simulink model "IndustrialMicrogrid"  (R2023a)
settings: Solver=FixedStepDiscrete  StartTime=0.0  StopTime=10  FixedStep=Ts  RelTol=1e-3
PostLoadFcn:
  | IndustrialMicrogridInputData
  | GfmGridFormingConverterInputParameters
model workspace (MAT data in the model file):
  caseNum = 2
undefined symbols (not defined in the file): base, BESS, DiscIntNeverNeededParam, grid, Grid, gridInverter, machine, microgrid, PV, PVInverter, PVTransformer, scrFactorRg, scrFactorXg, transformer, Ts
libraries: ee_lib x112, eeGeneralControl x104, nesl_utility_internal x64, simulink x56, nesl_utility x37, fl_lib x29, slpidlib x13, eeTransforms x11, eeTotalHarmonicDistorsion x8, eeRmsMeasurement x4, eeSinusoidalMeasurement x4, simulink_extras x2
(part 5 of 14)

== system IndustrialMicrogrid/MG1 Primary Substation/Microgrid Controller/Breaker Control ==
  Bus Element In1 : Inport  PortName=Control Room  Element=ResynchCmd
  Bus Element In4 : Inport  PortName=Control Room  Element=BRKcontrol
  Bus Element In6 : Inport  PortName=Control Room  Element=BRKcontrol
  Bus Element In3 : Inport  PortName=Control Room  Element=PlannedIslandCmd
  Bus Element In5 : Inport  Port=2  PortName=MGController  Element=IslandMGController.MGPlannedIsland.plannedisland
  Bus Element In2 : Inport  Port=2  PortName=MGController  Element=ResynchMGController.MGResynch.resynch
  Cast To Double1 : DataTypeConversion  OutDataTypeStr=double  SaturateOnIntegerOverflow=off  RndMeth=Floor
  Logical Operator1 : Logic  Operator=NOT  AllPortsSameDT=off  OutDataTypeStr=boolean
  Logical Operator{2..5} (4 alike) : Logic  AllPortsSameDT=off  OutDataTypeStr=boolean
  Logical Operator6 : Logic  Operator=OR  AllPortsSameDT=off  OutDataTypeStr=boolean
  Logical Operator7 : Logic  Operator=NOT  AllPortsSameDT=off  OutDataTypeStr=boolean
  BreakerControl : Outport
  wires:
  Logical Operator7/1 -> Logical Operator5/1
  Logical Operator1/1 -> Logical Operator4/1
  Logical Operator5/1 -> Logical Operator6/2
  Logical Operator3/1 -> Logical Operator4/2
  Bus Element In6/1 -> Logical Operator1/1
  Logical Operator6/1 -> Cast To Double1/1
  Bus Element In5/1 -> Logical Operator3/2
  Bus Element In4/1 -> Logical Operator5/2
  Logical Operator4/1 -> Logical Operator6/1
  Bus Element In1/1 -> Logical Operator2/1
  Logical Operator2/1 -> Logical Operator7/1
  Cast To Double1/1 -> BreakerControl/1
  Bus Element In3/1 -> Logical Operator3/1
  Bus Element In2/1 -> Logical Operator2/2

== system IndustrialMicrogrid/MG1 Primary Substation/Microgrid Controller/Frequency Reference ==
  Bus Element In : Inport  PortName=Control Room  Element=ResynchCmd
  Bus Element In1 : Inport  PortName=Control Room  Element=PowerCmd
  Bus Element In4 : Inport  PortName=Control Room  Element=BlackStartMG1
  Bus Element In2 : Inport  Port=2  PortName=MGController  Element=ResynchMGController.MGResynch.synchfrequency
  Bus Element In3 : Inport  Port=2  PortName=MGController  Element=BlackStart.Fref1
  Constant : Constant  Value=IslandFrequency
  Constant1 : Constant  Value=GridFrequency
  Gain1 : Gain  Gain=1/60
  Sum : Sum  Inputs=|++
  Switch : Switch  Criteria=u2 > Threshold  Threshold=0.5  SaturateOnIntegerOverflow=off  InputSameDT=off
  Switch1 : Switch  Criteria=u2 > Threshold  Threshold=0.5  SaturateOnIntegerOverflow=off  InputSameDT=off
  Switch2 : Switch  Criteria=u2 > Threshold  Threshold=0.5  SaturateOnIntegerOverflow=off  InputSameDT=off
  fref : Outport
  wires:
  Bus Element In/1 -> Switch/2
  Switch2/1 -> Switch1/3
  Bus Element In2/1 -> Sum/1
  Switch1/1 -> Gain1/1
  Bus Element In3/1 -> Switch1/1
  Gain1/1 -> fref/1
  Bus Element In4/1 -> Switch1/2
  Bus Element In1/1 -> Switch2/2
  Constant/1 -> Switch/3, Sum/2
  Sum/1 -> Switch/1
  Constant1/1 -> Switch2/1
  Switch/1 -> Switch2/3

== system IndustrialMicrogrid/MG1 Primary Substation/Microgrid Controller/PLL ==
  In Bus Element : Inport  PortName=mPCC  Element=Grid voltage
  In Bus Element1 : Inport  PortName=mPCC  Element=mPCC.voltage
  PLL : Subsystem
  PLL start at 0.2 s : Subsystem
  PLL starts at 0.2 s : Subsystem
  PLL1 : Subsystem
  Bus Element Out : Outport  PortName=Grid  Element=frequency
  Bus Element Out1 : Outport  PortName=Grid  Element=angle
  Bus Element Out2 : Outport  PortName=Grid  Element=voltage
  Bus Element Out3 : Outport  Port=2  PortName=Island  Element=voltage
  Bus Element Out4 : Outport  Port=2  PortName=Island  Element=frequency
  Bus Element Out5 : Outport  Port=2  PortName=Island  Element=angle
  wires:
  In Bus Element/1 -> PLL start at 0.2 s/1(PCC measurement)
  PLL starts at 0.2 s/1(abc) -> PLL1/1(abc)
  In Bus Element1/1 -> PLL starts at 0.2 s/1(PCC measurement)
  PLL start at 0.2 s/1(Out1) -> PLL/1(abc)
  PLL/1(fre) -> Bus Element Out/1
  PLL/2(angle) -> Bus Element Out1/1
  PLL/3(mag) -> Bus Element Out2/1
  PLL1/1(fre) -> Bus Element Out4/1
  PLL1/2(angle) -> Bus Element Out5/1
  PLL1/3(mag) -> Bus Element Out3/1

== system IndustrialMicrogrid/MG1 Primary Substation/Microgrid Controller/Planned Island ==
  mPCCPLL : Inport
  Control Room : Inport  Port=2
  Bus Creator : BusCreator  Inputs=2
  Control for Zero Powerflow : Subsystem  mask(Planned Island Control){KpPPlannedIsland=microgrid.KpPPlannedIsland, KiPPlannedIsland=microgrid.KiPPlannedIsland, KpQPlannedIsland=microgrid.KpQPlannedIsland, KiQPlannedIsland=microgrid.KiQPlannedIsland, ZeroActivePowerThreshold=microgrid.zeroActivePowerThreshold, ZeroReactivePowerThreshold=microgrid.zeroReactivePowerThreshold, PlannedIslandDelay=microgrid.plannedIslandDelay}
      mask prompts: KpPPlannedIsland "Active Power Planned Island Proportional Gain"; KiPPlannedIsland "Active Power Planned Island Integral Gain"; KpQPlannedIsland "Reactive Power Planned Island Proportional Gain"; KiQPlannedIsland "Reactive Power Planned Island Intergal Gain"; ZeroActivePowerThreshold "Zero Active Power Threshold"; ZeroReactivePowerThreshold "Zero Reactive Power Threshold"; PlannedIslandDelay "Planned Island Delay"
      mask help: provide planned island control parameters
  IslandMGController : Outport
  wires:
  mPCCPLL/1 -> Bus Creator/2, Control for Zero Powerflow/2(mPCCPLL)  "PCC measurments"
  Control for Zero Powerflow/1(MGController) -> Bus Creator/1  "MGPlannedIsland"
  Bus Creator/1 -> IslandMGController/1  "IslandMGController"
  Control Room/1 -> Control for Zero Powerflow/1(ControlRoom)

== system IndustrialMicrogrid/MG1 Primary Substation/Microgrid Controller/Resynchronization ==
  Control Room : Inport
  mPCCPLL : Inport  Port=2
  BESS : Inport  Port=3
  Bus Creator : BusCreator  Inputs=2
  Frequency and voltage matching : Subsystem  mask(Resynchronization Control){GridFrequency=grid.frequency, RadToDegree=microgrid.radToDegree, KpFreResynch=microgrid.KpFreResynch, KiFreResynch=microgrid.KiFreResynch, KpVolResynch=microgrid.KpVolResynch, KiVolResynch=microgrid.KiVolResynch, KpAngResynch=microgrid.KpAngResynch, KiAngResynch=microgrid.KiAngResynch, FrequencyThreshold=microgrid.frequencyThreshold, AngleThreshold=microgrid.angleThreshold, VoltageThreshold=microgrid.voltageThreshold, ResynchDelay=microgrid.resynchDelay, kDroop=microgrid.KDroop}
      mask prompts: GridFrequency "Grid Frequency"; RadToDegree "Rad to Degree"; KpFreResynch "Frequency Resynch Proportional Gain"; KiFreResynch "Frequency Resynch Integral Gain"; KpVolResynch "Voltage Resynch Proportional Gain"; KiVolResynch "Voltage Resynch Integral Gain"; KpAngResynch "Angle Resynch Proportional Gain"; KiAngResynch "Angle Resynch Integral Gain"; FrequencyThreshold "Frequency Matching Threshold"; AngleThreshold "Angle Matching Threshold"; VoltageThreshold "Voltage Matching Threshold"; ResynchDelay "Resynch Delay"; kDroop "Voltage Droop"
      mask help: Provide input for resynchronization control parameters
  ResynchMGController : Outport
  wires:
  Control Room/1 -> Frequency and voltage matching/2(ControlRoom)
  Bus Creator/1 -> ResynchMGController/1  "ResynchMGController"
  Frequency and voltage matching/1(MGController) -> Bus Creator/1  "MGResynch"
  BESS/1 -> Frequency and voltage matching/1(BESS)
  mPCCPLL/1 -> Bus Creator/2, Frequency and voltage matching/3(mPCCPLL)  "PCC measurments"

== system IndustrialMicrogrid/MG1 Primary Substation/Microgrid Controller/Voltage Reference ==
  Bus Element In1 : Inport  PortName=Control Room  Element=ResynchCmd
  Bus Element In2 : Inport  PortName=Control Room  Element=BlackStartMG1
  Bus Element In3 : Inport  Port=2  PortName=MGController  Element=ResynchMGController.MGResynch.synchvoltagedpr
  Bus Element In4 : Inport  Port=2  PortName=MGController  Element=BlackStart.Vref1
  Constant9 : Constant  Value=IslandVoltage
  Switch1 : Switch  Criteria=u2 > Threshold  Threshold=0.5  SaturateOnIntegerOverflow=off  InputSameDT=off
  Switch2 : Switch  Criteria=u2 > Threshold  Threshold=0.5  SaturateOnIntegerOverflow=off  InputSameDT=off
  Vref : Outport
  wires:
  Switch2/1 -> Vref/1
  Switch1/1 -> Switch2/3
  Bus Element In2/1 -> Switch2/2
  Constant9/1 -> Switch1/3
  Bus Element In1/1 -> Switch1/2
  Bus Element In4/1 -> Switch2/1
  Bus Element In3/1 -> Switch1/1

== system IndustrialMicrogrid/MG1 Primary Substation/PCC Measurements and PCC Breaker/Grid Current Measurement ==
  Current and Voltage Sensor (Three-Phase)1 : ee_lib/Sensors & Transducers/Current and Voltage Sensor (Three-Phase)  vMeasurementType=ee.enum.vmeasurement.ll  outputUnit=ee.enum.unit.pu  SRated=2.5e6 A*V  VRated=microgrid.voltage V  I_specify=off  I_priority=None  I=[0, 0, 0] A  I_nominal_specify=off  I_nominal_unit=A  I_nominal_value=1  V_specify=off  V_priority=None  V=[0, 0, 0] V  V_nominal_specify=off  V_nominal_unit=V  V_nominal_value=1
      settings: InternalSimscapePortConfiguration="{\"Bottom\":[],\"Left\":[{\"id\":\"N1\",\"label\":\"~1\",\"type\":\"foundation.electrical.three_phase\"}],\"Right\":[{\"id\":\"V_output\",\"label\":\"V\",\"type\":\"output\"},{\"id\":\"I_output\",\"label\":\"I\",\"type\":\"output\"},{\"id\":\"N2\",\"label\":\"~2\",\"type\":\"foundation.electrical.three_phase\"}],\"Top\":[]}"
  PS-Simulink Converter2 : nesl_utility_internal/PS-Simulink Converter  PhysicalDomain=network_engine_domain  SubClassName=ps_output  LeftPortType=input  RightPortType=output  PseudoPeriodic=off  Frequencies=[]  VectorFormat=1-D array  Unit=V  AffineConversion=off
  PS-Simulink Converter3 : nesl_utility_internal/PS-Simulink Converter  PhysicalDomain=network_engine_domain  SubClassName=ps_output  LeftPortType=input  RightPortType=output  PseudoPeriodic=off  Frequencies=[]  VectorFormat=1-D array  Unit=A  AffineConversion=off
  Terminator : Terminator
  ~ : PMIOPort  Side=Left
  "~ " : PMIOPort  Port=2  Side=Right
  "Grid voltage " : Outport
  wires:
  PS-Simulink Converter2/1 -> "Grid voltage "/1
  PS-Simulink Converter3/1 -> Terminator/1
  connections:
  Current and Voltage Sensor (Three-Phase)1/RConn1 -- PS-Simulink Converter2/LConn1
  ~/RConn1 -- Current and Voltage Sensor (Three-Phase)1/LConn1
  Current and Voltage Sensor (Three-Phase)1/RConn2 -- PS-Simulink Converter3/LConn1
  Current and Voltage Sensor (Three-Phase)1/RConn3 -- "~ "/RConn1

== system IndustrialMicrogrid/MG1 Primary Substation/PCC Measurements and PCC Breaker/Grid Power Measurement ==
  Current and Voltage Sensor (Three-Phase) : ee_lib/Sensors & Transducers/Current and Voltage Sensor (Three-Phase)  vMeasurementType=ee.enum.vmeasurement.ll  outputUnit=ee.enum.unit.pu  SRated=2.5e6 A*V  VRated=microgrid.voltage V  I_specify=off  I_priority=None  I=[0, 0, 0] A  I_nominal_specify=off  I_nominal_unit=A  I_nominal_value=1  V_specify=off  V_priority=None  V=[0, 0, 0] V  V_nominal_specify=off  V_nominal_unit=V  V_nominal_value=1
      settings: InternalSimscapePortConfiguration="{\"Bottom\":[],\"Left\":[{\"id\":\"N1\",\"label\":\"~1\",\"type\":\"foundation.electrical.three_phase\"}],\"Right\":[{\"id\":\"V_output\",\"label\":\"V\",\"type\":\"output\"},{\"id\":\"I_output\",\"label\":\"I\",\"type\":\"output\"},{\"id\":\"N2\",\"label\":\"~2\",\"type\":\"foundation.electrical.three_phase\"}],\"Top\":[]}"
  Low-Pass Filter (Discrete or Continuous) : eeGeneralControl/Low-Pass Filter (Discrete or Continuous)  K=1  T=0.1  B=inf  A=-inf  init_option=Inherited from block input  x0=0  Ts=Ts
  Low-Pass Filter (Discrete or Continuous)1 : eeGeneralControl/Low-Pass Filter (Discrete or Continuous)  K=1  T=0.1  B=inf  A=-inf  init_option=Inherited from block input  x0=0  Ts=Ts
  PS-Simulink Converter : nesl_utility_internal/PS-Simulink Converter  PhysicalDomain=network_engine_domain  SubClassName=ps_output  LeftPortType=input  RightPortType=output  PseudoPeriodic=off  Frequencies=[]  VectorFormat=1-D array  Unit=inherit  AffineConversion=off
  PS-Simulink Converter1 : nesl_utility_internal/PS-Simulink Converter  PhysicalDomain=network_engine_domain  SubClassName=ps_output  LeftPortType=input  RightPortType=output  PseudoPeriodic=off  Frequencies=[]  VectorFormat=1-D array  Unit=inherit  AffineConversion=off
  PS-Simulink Converter8 : nesl_utility_internal/PS-Simulink Converter  PhysicalDomain=network_engine_domain  SubClassName=ps_output  LeftPortType=input  RightPortType=output  PseudoPeriodic=off  Frequencies=[]  VectorFormat=1-D array  Unit=MW  AffineConversion=off
  PS-Simulink Converter9 : nesl_utility_internal/PS-Simulink Converter  PhysicalDomain=network_engine_domain  SubClassName=ps_output  LeftPortType=input  RightPortType=output  PseudoPeriodic=off  Frequencies=[]  VectorFormat=1-D array  Unit=MV*A  AffineConversion=off
  Power Sensor (Three-Phase)2 : ee_lib/Sensors & Transducers/Power Sensor (Three-Phase)  load_type=ee.enum.passive.type_balanced.balanced  f0=60 Hz  config=ee.enum.with_neutral.no  rho=1
      settings: InternalSimscapePortConfiguration="{\"Bottom\":[],\"Left\":[{\"id\":\"N1\",\"label\":\"~1\",\"type\":\"foundation.electrical.three_phase\"}],\"Right\":[{\"id\":\"N2\",\"label\":\"~2\",\"type\":\"foundation.electrical.three_phase\"}],\"Top\":[{\"id\":\"Pm\",\"label\":\"P\",\"type\":\"output\"},{\"id\":\"Qm\",\"label\":\"Q\",\"type\":\"output\"}]}"
  ~ : PMIOPort  Side=Left
  "~ " : PMIOPort  Port=2  Side=Right
  Out Bus Element : Outport  PortName=mPCC  Element=voltage
  Out Bus Element1 : Outport  PortName=mPCC  Element=current
  Out Bus Element2 : Outport  PortName=mPCC  Element=activepower
  Out Bus Element3 : Outport  PortName=mPCC  Element=reactivepower
  wires:
  PS-Simulink Converter8/1 -> Low-Pass Filter (Discrete or Continuous)/1
  PS-Simulink Converter9/1 -> Low-Pass Filter (Discrete or Continuous)1/1
  PS-Simulink Converter/1 -> Out Bus Element/1
  PS-Simulink Converter1/1 -> Out Bus Element1/1
  Low-Pass Filter (Discrete or Continuous)/1 -> Out Bus Element2/1
  Low-Pass Filter (Discrete or Continuous)1/1 -> Out Bus Element3/1
  connections:
  Current and Voltage Sensor (Three-Phase)/RConn2 -- PS-Simulink Converter1/LConn1
  PS-Simulink Converter/LConn1 -- Current and Voltage Sensor (Three-Phase)/RConn1
  Power Sensor (Three-Phase)2/RConn1 -- Current and Voltage Sensor (Three-Phase)/LConn1
  PS-Simulink Converter9/LConn1 -- Power Sensor (Three-Phase)2/LConn3
  Current and Voltage Sensor (Three-Phase)/RConn3 -- "~ "/RConn1
  PS-Simulink Converter8/LConn1 -- Power Sensor (Three-Phase)2/LConn2
  ~/RConn1 -- Power Sensor (Three-Phase)2/LConn1

== system IndustrialMicrogrid/MG2 PV Plant/(500KWp PV)/Measurement2 ==
  u : Inport
  Lead-Lag (Discrete or Continuous) : eeGeneralControl/Lead-Lag (Discrete or Continuous)  T1=0  T2=PV.controllerTSensor  B=inf  A=-inf  init_option=Inherited from block input  x0=0  Ts=Ts
      settings: LibrarySourceBlock=|
      | ee_sl_lib/General Control/Lead-Lag
      | (Discrete or Continuous)
  Out Bus Element : Outport  PortName=ipv1  Element=1
  wires:
  Lead-Lag (Discrete or Continuous)/1 -> Out Bus Element/1
  u/1 -> Lead-Lag (Discrete or Continuous)/1

== system IndustrialMicrogrid/MG2 PV Plant/(500KWp PV)/PV Inverter A2 ==
  note: Voltage reference for the PV inverter
  Insolation : Inport
  In Bus Element : Inport  Port=2  PortName=Vbus
  In Bus Element2 : Inport  Port=3  PortName=LVRT
  In Bus Element1 : Inport  Port=4  PortName=ipv1
  Q_ref : Inport  Port=5
  PV & Inverter : Subsystem
  PV Controller : Subsystem
  abc : PMIOPort  Side=Right
  wires:
  Q_ref/1 -> PV Controller/5(Q_ref)
  PV Controller/1(m_abc) -> [m]
  In Bus Element1/1 -> PV Controller/2(ipv1)
  PV & Inverter/1(PV_plant1) -> PV Controller/1(PV_plant1)
  In Bus Element/1 -> PV Controller/4(Vbus)
  In Bus Element2/1 -> PV Controller/3(LVRT)
  [m] -> PV & Inverter/2(reference)
  Insolation/1 -> PV & Inverter/1(Solar insolation)
  connections:
  abc/RConn1 -- PV & Inverter/RConn1

== system IndustrialMicrogrid/MG2 PV Plant/PLL & Measurements2/Measurement2 ==
  u : Inport
  Lead-Lag Filter1 : spsLeadLagFilterLib/Lead-Lag Filter  T1=0  T2=PV.controllerTSensor  Vdc_Init=0  Ts=Ts
  Vg : Outport
  wires:
  Lead-Lag Filter1/1 -> Vg/1
  u/1 -> Lead-Lag Filter1/1

== system IndustrialMicrogrid/MG2 PV Plant/PLL & Measurements2/PLL ==
  abc : Inport
  Demux : Demux  Outputs=3
  Park Transform : eeTransforms/Park Transform  AxisAlignment=Q-axis  PowerInvariant=off
  "Sinusoidal Measurement (PLL, Three-Phase)" : eeSinusoidalMeasurementV2/Sinusoidal Measurement (PLL, Three-Phase)  Kp_LF=PV.kpPLL  Ki_LF=PV.kiPLL  F0=60  Theta0=0  Ts=-1
      settings: LibrarySourceBlock=|
      | ee_sl_lib/Measurements/Sinusoidal Measurement
      | (PLL, Three-Phase)
  Terminator : Terminator
  mag : Outport
  freq : Outport  Port=2
  angle : Outport  Port=3
  Vd : Outport  Port=4
  Vq : Outport  Port=5
  wires:
  Demux/3 -> Terminator/1
  abc/1 -> Park Transform/1, "Sinusoidal Measurement (PLL, Three-Phase)"/1
  Park Transform/1 -> Demux/1
  Demux/1 -> Vd/1
  Demux/2 -> Vq/1
  "Sinusoidal Measurement (PLL, Three-Phase)"/2 -> Park Transform/2, angle/1
  "Sinusoidal Measurement (PLL, Three-Phase)"/1 -> freq/1
  "Sinusoidal Measurement (PLL, Three-Phase)"/3 -> mag/1

== system IndustrialMicrogrid/MG2 Power Center/Diesel Generator/AVR and Exciter ==
  Constant{3,5..9} (6 alike) : Constant  Value=0
  Constant4 : Constant  Value=1.08
  "E_FD Simulink-PS " : nesl_utility/Simulink-PS Converter  PhysicalDomain=network_engine_domain  SubClassName=ps_input  LeftPortType=input  RightPortType=output  PseudoPeriodic=off  Frequencies=[]  NoiseDistribution=none  NoiseParameters=[]  Unit=1  AffineConversion=off  FilteringAndDerivatives=provide  SimscapeFilterOrder=1  InputFilterTimeConstant=.001  UdotUserProvided=0
  I_FD PS-Simulink : nesl_utility/PS-Simulink Converter  PhysicalDomain=network_engine_domain  SubClassName=ps_output  LeftPortType=input  RightPortType=output  PseudoPeriodic=off  Frequencies=[]  VectorFormat=1-D array  Unit=1  AffineConversion=off
  SM DC2C : eeSmDC2C/SM DC2C  E_FD0=1  Ts=-1  R_C=0  X_C=0  T_R=0  K_A=300  T_A=0.06  T_B=0  T_C=0  K_F=0.058  T_F=0.62  V_Rmax=4.5  V_Rmin=-4.5  oelInputLocation=Unused  uelInputLocation=Unused  sclInputLocation=Unused  K_E=1  T_E=1.33  E_FDmin=-99  E_1=3.05  S_E_E1=0.279  E_2=2.29  S_E_E2=0.117
  Synchronous Machine Field Circuit (pu) : ee_lib/Electromechanical/Synchronous/Synchronous Machine Field Circuit  unit_option=ee.enum.unit.pu  SRated=microgrid.dieselRatedPower V*A  FRated=microgrid.frequency Hz  fieldCircuitParameterization_option=ee.enum.sm.fieldparameterization.current  baseEfd=200 V  baseIfd=1300 A  parameterization_option=2  Ladu=1.66  Rfd=0.0006  Xl=0.05  Xd=1.72  Xdd=0.13  Xddd=0.09  d_option=ee.enum.circuit.open  Td0d=0.75 s  Tdd=0.03 s  Td0dd=0.003 s  Tddd=0.008 s
      settings: InternalSimscapePortConfiguration="{\"Bottom\":[],\"Left\":[{\"id\":\"Efd_pu\",\"label\":\"Efd_pu\",\"type\":\"input\"},{\"id\":\"Ifd_pu\",\"label\":\"Ifd_pu\",\"type\":\"output\"}],\"Right\":[{\"id\":\"fd_p\",\"label\":\"fd+\",\"type\":\"foundation.electrical.electrical\"},{\"id\":\"fd_n\",\"label\":\"fd-\",\"type\":\"foundation.electrical.electrical\"}],\"Top\":[]}"
  Terminal Current Measurement : ee_lib/Electromechanical/Synchronous/Synchronous Machine Measurement  output_idx=15
      settings: InternalSimscapePortConfiguration="{\"Bottom\":[],\"Left\":[{\"id\":\"pu_input\",\"label\":\"pu\",\"type\":\"input\"}],\"Right\":[{\"id\":\"pu_output\",\"label\":\"o\",\"type\":\"output\"}],\"Top\":[]}"
  Terminal Current PS-Simulink : nesl_utility/PS-Simulink Converter  PhysicalDomain=network_engine_domain  SubClassName=ps_output  LeftPortType=input  RightPortType=output  PseudoPeriodic=off  Frequencies=[]  VectorFormat=1-D array  Unit=1  AffineConversion=off
  Terminal Voltage Measurement : ee_lib/Electromechanical/Synchronous/Synchronous Machine Measurement  output_idx=14
      settings: InternalSimscapePortConfiguration="{\"Bottom\":[],\"Left\":[{\"id\":\"pu_input\",\"label\":\"pu\",\"type\":\"input\"}],\"Right\":[{\"id\":\"pu_output\",\"label\":\"o\",\"type\":\"output\"}],\"Top\":[]}"
  Terminal Voltage PS-Simulink : nesl_utility/PS-Simulink Converter  PhysicalDomain=network_engine_domain  SubClassName=ps_output  LeftPortType=input  RightPortType=output  PseudoPeriodic=off  Frequencies=[]  VectorFormat=1-D array  Unit=1  AffineConversion=off
  Terminator : Terminator
  Unit Delay : UnitDelay  InitialCondition=1.32943  SampleTime=-1  HasFrameUpgradeWarning=on
  pu : PMIOPort  Side=Left
  fd+ : PMIOPort  Port=2  Side=Right
  fd- : PMIOPort  Port=3  Side=Right
  wires:
  Terminal Current PS-Simulink/1 -> SM DC2C/4
  SM DC2C/1 -> "E_FD Simulink-PS "/1
  Constant9/1 -> SM DC2C/9
  Constant8/1 -> SM DC2C/8
  Constant7/1 -> SM DC2C/7
  Constant6/1 -> SM DC2C/6
  Constant5/1 -> SM DC2C/5
  Constant4/1 -> SM DC2C/1
  Constant3/1 -> SM DC2C/2
  Terminal Voltage PS-Simulink/1 -> SM DC2C/3
  I_FD PS-Simulink/1 -> Unit Delay/1
  Unit Delay/1 -> Terminator/1
  connections:
  Terminal Current Measurement/RConn1 -- Terminal Current PS-Simulink/LConn1
  Terminal Voltage Measurement/RConn1 -- Terminal Voltage PS-Simulink/LConn1
  pu/RConn1 -- Terminal Current Measurement/LConn1 -- Terminal Voltage Measurement/LConn1
  Synchronous Machine Field Circuit (pu)/RConn1 -- fd+/RConn1
  fd-/RConn1 -- Synchronous Machine Field Circuit (pu)/RConn2
  I_FD PS-Simulink/LConn1 -- Synchronous Machine Field Circuit (pu)/LConn2
  "E_FD Simulink-PS "/RConn1 -- Synchronous Machine Field Circuit (pu)/LConn1

== system IndustrialMicrogrid/MG2 Power Center/Diesel Generator/Governor and Prime Mover  ==
  Governor : Subsystem
  Ideal Torque Source : fl_lib/Mechanical/Mechanical Sources/Ideal Torque Source
  Mechanical Rotational Reference : fl_lib/Mechanical/Rotational Elements/Mechanical Rotational Reference
  Non-reheat turbine : Subsystem
  PS-Simulink Converter : nesl_utility/PS-Simulink Converter  PhysicalDomain=network_engine_domain  SubClassName=ps_output  LeftPortType=input  RightPortType=output  PseudoPeriodic=off  Frequencies=[]  VectorFormat=1-D array  Unit=1  AffineConversion=off
  Rotor Velocity Measurement : ee_lib/Electromechanical/Synchronous/Synchronous Machine Measurement  output_idx=4
      settings: InternalSimscapePortConfiguration="{\"Bottom\":[],\"Left\":[{\"id\":\"pu_input\",\"label\":\"pu\",\"type\":\"input\"}],\"Right\":[{\"id\":\"pu_output\",\"label\":\"o\",\"type\":\"output\"}],\"Top\":[]}"
  Simulink-PS Converter : nesl_utility/Simulink-PS Converter  PhysicalDomain=network_engine_domain  SubClassName=ps_input  LeftPortType=input  RightPortType=output  PseudoPeriodic=off  Frequencies=[]  NoiseDistribution=none  NoiseParameters=[]  Unit=1  AffineConversion=off  FilteringAndDerivatives=zero  SimscapeFilterOrder=1  InputFilterTimeConstant=0.001  UdotUserProvided=1
  scale by base_torque : Gain  Gain=base_torque
  R : PMIOPort  Side=Right
  C : PMIOPort  Port=2  Side=Right
  pu : PMIOPort  Port=3  Side=Left
  wires:
  PS-Simulink Converter/1 -> Governor/1(pu_velocity)
  Governor/1(delta_y) -> Non-reheat turbine/1(delta_y)
  Non-reheat turbine/1(torque) -> scale by base_torque/1
  scale by base_torque/1 -> Simulink-PS Converter/1
  connections:
  C/RConn1 -- Ideal Torque Source/RConn2 -- Mechanical Rotational Reference/LConn1
  Ideal Torque Source/LConn1 -- R/RConn1
  pu/RConn1 -- Rotor Velocity Measurement/LConn1
  PS-Simulink Converter/LConn1 -- Rotor Velocity Measurement/RConn1
  Simulink-PS Converter/RConn1 -- Ideal Torque Source/RConn1

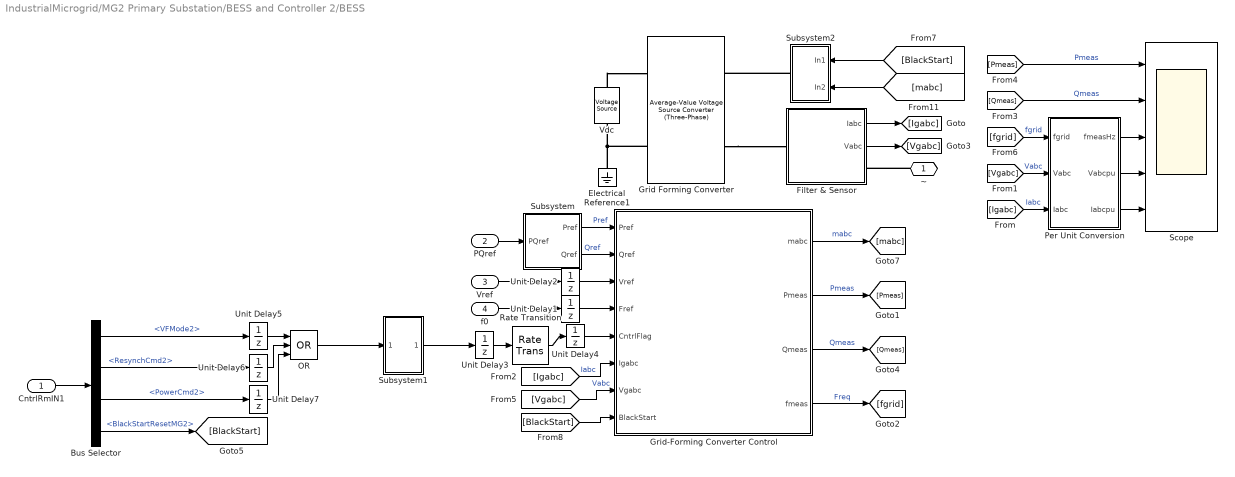
== system IndustrialMicrogrid/MG2 Primary Substation/BESS and Controller 2/BESS ==
  CntrlRmIN1 : Inport
  PQref : Inport  Port=2
  Vref : Inport  Port=3
  f0 : Inport  Port=4
  Bus Selector : BusSelector  OutputSignals=VFMode2,ResynchCmd2,PowerCmd2,BlackStartResetMG2
  Electrical Reference1 : fl_lib/Electrical/Electrical Elements/Electrical Reference
  Filter & Sensor : Subsystem
      mask Display: image('$imagefile'); % Use "Edit Image" on toolstrip to change.
  Grid Forming Converter : ee_lib/Semiconductors & Converters/Converters/Average-Value Voltage Source Converter (Three-Phase)  port_option=ee.enum.threePhasePort.composite  frequency_option=ee.enum.converters.frequency.variable  FRated=50 Hz  losses_parameterization=ee.enum.converters.losses.fixed  Pfixed=1 W  ks=0.01  kc1=1.7 V  kc2=0.01 Ohm  Ploss_vect=[100, 800, 1870, 3250, 4900] W  Irms_vect=[10, 100, 200, 300, 400] A  Vdc_nom=300 V  thermal_mass=30000 J/K  temperature_specify=off  temperature_priority=High  temperature=298.15 K  temperature_nominal_specify=off  temperature_nominal_unit=K  temperature_nominal_value=1
      settings: InternalSimscapePortConfiguration="{\"Bottom\":[],\"Left\":[{\"id\":\"ModWave\",\"label\":\"ModWave\",\"type\":\"input\"},{\"id\":\"N\",\"label\":\"~\",\"type\":\"foundation.electrical.three_phase\"}],\"Right\":[{\"id\":\"p\",\"label\":\"+\",\"type\":\"foundation.electrical.electrical\"},{\"id\":\"n\",\"label\":\"-\",\"type\":\"foundation.electrical.electrical\"}],\"Top\":[]}"
  Grid-Forming Converter Control : Subsystem  mask(Grid Forming Controller){power=gridInverter.apparentPower*1e3, girdLineVoltage=gridInverter.lineRMSVoltage, powerFreq=gridInverter.frequency, dcBusVoltage=gridInverter.DCVoltage, measSampleTime=gridInverter.measurementSampleTime, powerControl=Virtual Synchronous Machine, activePowerSampleTime=gridInverter.droopControl.sampleTime, droopSlope=gridInverter.droopControl.freqSlopeMp, droopT1=gridInverter.droopControl.T1, droopT2=gridInverter.droopControl.T2, droopTC=gridInverter.droopControl.lpfTimeConst, vsmPmeasFilterTC=gridInverter.vsm.PmeasTimeConst, vsmFreqDroop=gridInverter.vsm.freqDroop, vsmInertiaTC=gridInverter.vsm.inertiaConstant, vsmDampingConst=gridInverter.vsm.dampingCoefficent, dampingPowerMaxLimit=gridInverter.vsm.maxDampingPower, dampingPowerMinLimit=gridInverter.vsm.minDampingPower, freqMeasTimeConst=gridInverter.freqMeasTimeConst, freqOption=Constant Frequency Reference, voltreference=gridInverter.Qcontrol.voltageReference, QVoltFilterTC=gridInverter.Qcontrol.QmeasTimeConst, QVoltDroop=gridInverter.Qcontrol.voltageDroop, currentLimit=Virtual Impedance, maxSatCurrentLimit=gridInverter.currentLimit.maxSaturationCurrent, maxVICurrentLimit=gridInverter.currentLimit.viCurrentLimit, ctLimitVirtualImp=gridInverter.currentLimit.virImpResistanceCoeff, ctLimitXbyR=gridInverter.currentLimit.virImpXbyR, ctLimitDelayTime=gridInverter.currentLimit.maxSaturationDelay, currentSatTime=gridInverter.currentLimit.satCurrentRunTime, currentVITimeConst=gridInverter.currentLimit.viFilterTimeConst, voltControlTs=gridInverter.controller.VoltageControlSampleTime, vdPGain=gridInverter.controller.voltControllerKp, VdIGain=gridInverter.controller.voltControllerKi, VdMaxCt=gridInverter.controller.voltageMaxId, VdMinCt=gridInverter.controller.voltageMinId, VqPGain=gridInverter.controller.voltControllerKp, VqIGain=gridInverter.controller.voltControllerKi, VqMaxCt=gridInverter.controller.voltageMaxIq, VqMinCt=gridInverter.controller.voltageMinIq, vdvqLPFTimeConst=gridInverter.controller.voltMeasTimeConst, currentControlTs=gridInverter.controller.CurrentControlSampleTime, filterInductance=gridInverter.L, IdPGain=gridInverter.controller.ctControllerKp, IdIGain=gridInverter.controller.ctControllerKi, IqPGain=gridInverter.controller.ctControllerKp, IqIGain=gridInverter.controller.ctControllerKi}
      mask prompts: power "Grid forming converter power (VA)"; girdLineVoltage "Grid line voltage (V)"; powerFreq "Grid frequency (Hz)"; dcBusVoltage "DC bus voltage"; measSampleTime "Measurement sample time"; powerControl "Active Power Control"; activePowerSampleTime "Sample time (s)"; droopSlope "Power droop slope (pu, Hz/W)"; droopT1 "Lead-Lag numerator time constant (s)"; droopT2 "Lead-Lag denominator time constant (s)"; droopTC "Filter cut-off time constant (s)"; vsmPmeasFilterTC "Power measurement filter time constant (s)"; vsmFreqDroop "Frequency droop (pu,  W/Hz)"; vsmInertiaTC "Inertia constant M (pu)"; vsmDampingConst "Damping constant (pu/Hz)"; dampingPowerMaxLimit "Damping power maximum limit (pu)"; dampingPowerMinLimit "Damping power minimum limit (pu)"; freqMeasTimeConst "Frequency measurement time constant (s)"; freqOption "Damping power fequency option"; voltreference "Voltage reference value (pu)"; QVoltFilterTC "Power measurement filter time constant (s)"; QVoltDroop "Voltage droop (pu, V/VAR)"; currentLimit "Current limiting method"; maxSatCurrentLimit "Maximum current saturation (pu)"; maxVICurrentLimit "Maximum virtual impedance current (pu)"; ctLimitVirtualImp "Virtual impedance coefficient (pu.Ohm/pu.A)"; ctLimitXbyR "Virtual X/R ratio"; ctLimitDelayTime "Maximum current delay time (s)"; currentSatTime "Current limiting run time (s)"; currentVITimeConst "Filter time constant (s)"; voltControlTs "Controller sample time (s)"; vdPGain "Vd proportional gain"; VdIGain "Vd integral gain"; VdMaxCt "Vd maximum current limit (A)"; VdMinCt "Vd minimum current limit (A)"; VqPGain "Vq proportional gain"; VqIGain "Vq integral gain"; VqMaxCt "Vq maximum current limit (A)"; VqMinCt "Vq minimum current limit (A)"; vdvqLPFTimeConst "Voltage measurement filter time constant (s)"; currentControlTs "Controller sample time (s)"; filterInductance "Filter inductance (H)"; IdPGain "Id proportional gain"; IdIGain "Id integral gain"; IqPGain "Iq proportional gain"; IqIGain "Iq integral gain"
      mask help: This block implements the grid forming controller with fault ride through capability. Input to the controller are active and reactive power reference in per unit and the sensed three-phase phase current in amphere and phase voltage in volts.
      mask init: same as IndustrialMicrogrid/MG1 Primary Substation/BESS and Controller/BESS/Grid-Forming Converter Control
      mask TypeOptions powerControl: Virtual Synchronous Machine | Droop Control
      mask Callback powerControl:
      | h = Simulink.Mask.get(gcb);
      | slectedActivePowerControl=get_param(gcb,'powerControl');
      | %slectedActivePowerControl = h.Parameters(find(string({h.Parameters.Name}) == 'powerControl')).Value;
      | switch slectedActivePowerControl
      |     case 'Virtual Synchronous Machine'
      |         h.Parameters(find(string({h.Parameters.Name}) == 'droopSlope')).Visible = 'off';
      |         h.Parameters(find(string({h.Parameters.Name}) == 'droopTC')).Visible = 'off';
      |         h.Parameters(find(string({h.Parameters.Name}) == 'droopT1')).Visible = 'off';
      |         h.Parameters(find(string({h.Parameters.Name}) == 'droopT2')).Visible = 'off';
      |         h.Parameters(find(string({h.Parameters.Name}) == 'vsmPmeasFilterTC')).Visible = 'on';
      |         h.Parameters(find(string({h.Parameters.Name}) == 'vsmFreqDroop')).Visible = 'on';
      |         h.Parameters(find(string({h.Parameters.Name}) == 'vsmInertiaTC')).Visible = 'on';
      |         h.Parameters(find(string({h.Parameters.Name}) == 'vsmDampingConst')).Visible = 'on';
      |         h.Parameters(find(string({h.Parameters.Name}) == 'dampingPowerMaxLimit')).Visible = 'on';
      |         h.Parameters(find(string({h.Parameters.Name}) == 'dampingPowerMinLimit')).Visible = 'on';
      |         h.Parameters(find(string({h.Parameters.Name}) == 'freqOption')).Visible = 'on';
      |         h.Parameters(find(string({h.Parameters.Name}) == 'freqMeasTimeConst')).Visible = 'on';
      |     case 'Droop Control'
      |         h.Parameters(find(string({h.Parameters.Name}) == 'droopSlope')).Visible = 'on';
      |         h.Parameters(find(string({h.Parameters.Name}) == 'droopTC')).Visible = 'on';
      |         h.Parameters(find(string({h.Parameters.Name}) == 'droopT1')).Visible = 'on';
      |         h.Parameters(find(string({h.Parameters.Name}) == 'droopT2')).Visible = 'on';
      |         h.Parameters(find(string({h.Parameters.Name}) == 'vsmPmeasFilterTC')).Visible = 'off';
      |         h.Parameters(find(string({h.Parameters.Name}) == 'vsmFreqDroop')).Visible = 'off';
      |         h.Parameters(find(string({h.Parameters.Name}) == 'vsmInertiaTC')).Visible = 'off';
      |         h.Parameters(find(string({h.Parameters.Name}) == 'vsmDampingConst')).Visible = 'off';
      |         h.Parameters(find(string({h.Parameters.Name}) == 'dampingPowerMaxLimit')).Visible = 'off';
      |         h.Parameters(find(string({h.Parameters.Name}) == 'dampingPowerMinLimit')).Visible = 'off';
      |         h.Parameters(find(string({h.Parameters.Name}) == 'freqOption')).Visible = 'off';
      |         h.Parameters(find(string({h.Parameters.Name}) == 'freqMeasTimeConst')).Visible = 'on';
      | 
      |     otherwise
      |         disp('Choose proper active power control method')
      | end
      mask TypeOptions freqOption: Use Grid Frequency Measurement | Constant Frequency Reference
      mask TypeOptions currentLimit: Virtual Impedance | Current Limiting | Combining Virtual Impedance and Current Limiting
      mask Callback currentLimit:
      | currentLimit = 1;
      | h = Simulink.Mask.get(gcb);
      | currentLimitControl=get_param(gcb,'currentLimit');
      | %slectedActivePowerControl = h.Parameters(find(string({h.Parameters.Name}) == 'powerControl')).Value;
      | switch currentLimitControl
      |     case 'Virtual Impedance'
      |         h.Parameters(find(string({h.Parameters.Name}) == 'maxVICurrentLimit')).Visible = 'on';
      |         h.Parameters(find(string({h.Parameters.Name}) == 'ctLimitVirtualImp')).Visible = 'on';
      |         h.Parameters(find(string({h.Parameters.Name}) == 'ctLimitXbyR')).Visible = 'on';
      |         h.Parameters(find(string({h.Parameters.Name}) == 'maxSatCurrentLimit')).Visible = 'off';
      |         h.Parameters(find(string({h.Parameters.Name}) == 'ctLimitDelayTime')).Visible = 'off';
      |         h.Parameters(find(string({h.Parameters.Name}) == 'currentSatTime')).Visible = 'off';
      |         h.Parameters(find(string({h.Parameters.Name}) == 'currentVITimeConst')).Visible = 'on';
      | 
      | 
      |     case 'Current Limiting'
      |         h.Parameters(find(string({h.Parameters.Name}) == 'maxVICurrentLimit')).Visible = 'off';
      |         h.Parameters(find(string({h.Parameters.Name}) == 'ctLimitVirtualImp')).Visible = 'off';
      |         h.Parameters(find(string({h.Parameters.Name}) == 'ctLimitXbyR')).Visible = 'off';
      |         h.Parameters(find(string({h.Parameters.Name}) == 'maxSatCurrentLimit')).Visible = 'on';
      |         h.Parameters(find(string({h.Parameters.Name}) == 'ctLimitDelayTime')).Visible = 'on';
      |         h.Parameters(find(string({h.Parameters.Name}) == 'currentSatTime')).Visible = 'off';
      |         h.Parameters(find(string({h.Parameters.Name}) == 'currentVITimeConst')).Visible = 'off';
      | 
      |     case 'Combining Virtual Impedance and Current Limiting'
      |         h.Parameters(find(string({h.Parameters.Name}) == 'maxVICurrentLimit')).Visible = 'on';
      |         h.Parameters(find(string({h.Parameters.Name}) == 'ctLimitVirtualImp')).Visible = 'on';
      |         h.Parameters(find(string({h.Parameters.Name}) == 'ctLimitXbyR')).Visible = 'on';
      |         h.Parameters(find(string({h.Parameters.Name}) == 'maxSatCurrentLimit')).Visible = 'on';
      |         h.Parameters(find(string({h.Parameters.Name}) == 'ctLimitDelayTime')).Visible = 'off';
      |         h.Parameters(find(string({h.Parameters.Name}) == 'currentSatTime')).Visible = 'on';
      |         h.Parameters(find(string({h.Parameters.Name}) == 'currentVITimeConst')).Visible = 'on';
      | 
      |     otherwise
      |         disp('Choose proper current limiting method')
      | end
      mask DialogControl ParameterGroupVar Prompt: Grid Forming Control Parameters
      mask DialogControl Container8 Prompt: Grid-forming Converter Specification
      mask DialogControl Pcontrolgrp Prompt: Active Power Controller Parameters
      mask DialogControl QcontrolGrp Prompt: Reactive Power Controller Parameters
      mask DialogControl faultRideThroughGrp Prompt: Fault Ride Through Parameters
      mask DialogControl voltControlgrp Prompt: Voltage Controller Parameters
      mask DialogControl Container15currentContGrp Prompt: Current Controller Parameters
      mask Display: image('$imagefile'); % Use "Edit Image" on toolstrip to change.
  OR : Logic  Operator=OR  Inputs=3  IconShape=distinctive  AllPortsSameDT=off  OutDataTypeStr=boolean
  Per Unit Conversion : Subsystem
  Rate Transition : RateTransition
  Scope : Scope  NumInputPorts=5
  Subsystem : Subsystem
  Subsystem1 : Subsystem
  Subsystem2 : Subsystem
  Unit Delay{1..4} (4 alike) : UnitDelay  InitialCondition=1  SampleTime=Ts  HasFrameUpgradeWarning=on
  Unit Delay5 : UnitDelay  SampleTime=Ts  HasFrameUpgradeWarning=on
  Unit Delay6 : UnitDelay  SampleTime=Ts  HasFrameUpgradeWarning=on
  Unit Delay7 : UnitDelay  SampleTime=Ts  HasFrameUpgradeWarning=on
  Vdc : ee_lib/Sources/Voltage Source  dc_voltage=gridInverter.DCVoltage V  ac_voltage=0 V  ac_shift=0 rad  ac_frequency=0 Hz  noise_mode=ee.enum.sources.noise.Disabled  PSD=0 V^2/Hz  sample_time=1e-3 s  repeatability=ee.enum.sources.repeatability.NotRepeatable  user_seed=0  auto_seed=3499211588  i_specify=off  i_priority=None  i=0 A  i_nominal_specify=off  i_nominal_unit=A  i_nominal_value=1  v_specify=off  v_priority=None  v=0 V  v_nominal_specify=off  v_nominal_unit=V  v_nominal_value=1
  "~ " : PMIOPort  Side=Left
  wires:
  Grid-Forming Converter Control/3(Qmeas) -> [Qmeas]  "Qmeas"
  Grid-Forming Converter Control/2(Pmeas) -> [Pmeas]  "Pmeas"
  Filter & Sensor/2(Vabc) -> [Vgabc]
  Filter & Sensor/1(Iabc) -> [Igabc]
  [Vgabc] -> Grid-Forming Converter Control/7(Vgabc)  "Vabc"
  Subsystem/1(Pref) -> Grid-Forming Converter Control/1(Pref)  "Pref"
  Grid-Forming Converter Control/1(mabc) -> [mabc]  "mabc"
  Subsystem/2(Qref) -> Grid-Forming Converter Control/2(Qref)  "Qref"
  [Igabc] -> Grid-Forming Converter Control/6(Igabc)  "Iabc"
  Per Unit Conversion/3(Iabcpu) -> Scope/5
  Per Unit Conversion/2(Vabcpu) -> Scope/4
  Per Unit Conversion/1(fmeasHz) -> Scope/3
  [Pmeas] -> Scope/1  "Pmeas"
  [Qmeas] -> Scope/2  "Qmeas"
  [Igabc] -> Per Unit Conversion/3(Iabc)  "Iabc"
  [fgrid] -> Per Unit Conversion/1(fgrid)  "fgrid"
  [Vgabc] -> Per Unit Conversion/2(Vabc)  "Vabc"
  Grid-Forming Converter Control/4(fmeas) -> [fgrid]  "Freq"
  CntrlRmIN1/1 -> Bus Selector/1
  PQref/1 -> Subsystem/1(PQref)
  Vref/1 -> Unit Delay2/1
  f0/1 -> Unit Delay1/1
  Subsystem1/1(Out1) -> Unit Delay3/1
  Rate Transition/1 -> Unit Delay4/1
  Unit Delay4/1 -> Grid-Forming Converter Control/5(CntrlFlag)
  Unit Delay3/1 -> Rate Transition/1
  Unit Delay1/1 -> Grid-Forming Converter Control/4(Fref)
  Unit Delay2/1 -> Grid-Forming Converter Control/3(Vref)
  Unit Delay7/1 -> OR/3
  Unit Delay6/1 -> OR/2
  Unit Delay5/1 -> OR/1
  OR/1 -> Subsystem1/1(In1)
  Bus Selector/1 -> Unit Delay5/1  "<VFMode2>"
  Bus Selector/2 -> Unit Delay6/1  "<ResynchCmd2>"
  Bus Selector/3 -> Unit Delay7/1  "<PowerCmd2>"
  Bus Selector/4 -> [BlackStart]  "<BlackStartResetMG2>"
  [BlackStart] -> Subsystem2/1(In1)
  [mabc] -> Subsystem2/2(In2)
  [BlackStart] -> Grid-Forming Converter Control/8(BlackStart)
  connections:
  Electrical Reference1/LConn1 -- Grid Forming Converter/RConn2 -- Vdc/RConn1
  "~ "/RConn1 -- Filter & Sensor/RConn1
  Grid Forming Converter/LConn2 -- Filter & Sensor/LConn1
  Vdc/LConn1 -- Grid Forming Converter/RConn1
  Subsystem2/RConn1 -- Grid Forming Converter/LConn1

== system IndustrialMicrogrid/MG2 Primary Substation/BESS and Controller 2/BESS Converter Measurement  ==
  Current and Voltage Sensor (Three-Phase) : ee_lib/Sensors & Transducers/Current and Voltage Sensor (Three-Phase)  vMeasurementType=ee.enum.vmeasurement.lg  outputUnit=ee.enum.unit.pu  SRated=1e6 A*V  VRated=microgrid.voltage V  I_specify=off  I_priority=None  I=[ 0 0 0 ] A  I_nominal_specify=off  I_nominal_unit=A  I_nominal_value=1  V_specify=off  V_priority=None  V=[ 0 0 0 ] V  V_nominal_specify=off  V_nominal_unit=V  V_nominal_value=1
      settings: InternalSimscapePortConfiguration="{\"Bottom\":[],\"Left\":[{\"id\":\"N1\",\"label\":\"~1\",\"type\":\"foundation.electrical.three_phase\"}],\"Right\":[{\"id\":\"V_output\",\"label\":\"V\",\"type\":\"output\"},{\"id\":\"I_output\",\"label\":\"I\",\"type\":\"output\"},{\"id\":\"N2\",\"label\":\"~2\",\"type\":\"foundation.electrical.three_phase\"}],\"Top\":[]}"
  Low-Pass Filter (Discrete or Continuous) : eeGeneralControl/Low-Pass Filter (Discrete or Continuous)  K=1  T=0.02  B=inf  A=-inf  init_option=Inherited from block input  x0=0  Ts=Ts
  Low-Pass Filter (Discrete or Continuous)1 : eeGeneralControl/Low-Pass Filter (Discrete or Continuous)  K=1  T=0.02  B=inf  A=-inf  init_option=Inherited from block input  x0=0  Ts=Ts
  PS-Simulink Converter2 : nesl_utility_internal/PS-Simulink Converter  PhysicalDomain=network_engine_domain  SubClassName=ps_output  LeftPortType=input  RightPortType=output  PseudoPeriodic=off  Frequencies=[]  VectorFormat=1-D array  Unit=V  AffineConversion=off
  PS-Simulink Converter3 : nesl_utility_internal/PS-Simulink Converter  PhysicalDomain=network_engine_domain  SubClassName=ps_output  LeftPortType=input  RightPortType=output  PseudoPeriodic=off  Frequencies=[]  VectorFormat=1-D array  Unit=A  AffineConversion=off
  PS-Simulink Converter6 : nesl_utility_internal/PS-Simulink Converter  PhysicalDomain=network_engine_domain  SubClassName=ps_output  LeftPortType=input  RightPortType=output  PseudoPeriodic=off  Frequencies=[]  VectorFormat=1-D array  Unit=MW  AffineConversion=off
  PS-Simulink Converter7 : nesl_utility_internal/PS-Simulink Converter  PhysicalDomain=network_engine_domain  SubClassName=ps_output  LeftPortType=input  RightPortType=output  PseudoPeriodic=off  Frequencies=[]  VectorFormat=1-D array  Unit=MV*A  AffineConversion=off
  Power Sensor (Three-Phase)1 : ee_lib/Sensors & Transducers/Power Sensor (Three-Phase)  load_type=ee.enum.passive.type_balanced.balanced  f0=60 Hz  config=ee.enum.with_neutral.no  rho=1
      settings: InternalSimscapePortConfiguration="{\"Bottom\":[],\"Left\":[{\"id\":\"N1\",\"label\":\"~1\",\"type\":\"foundation.electrical.three_phase\"}],\"Right\":[{\"id\":\"N2\",\"label\":\"~2\",\"type\":\"foundation.electrical.three_phase\"}],\"Top\":[{\"id\":\"Pm\",\"label\":\"P\",\"type\":\"output\"},{\"id\":\"Qm\",\"label\":\"Q\",\"type\":\"output\"}]}"
  a1 : PMIOPort  Side=Left
  ~ : PMIOPort  Port=2  Side=Right
  Out Bus Element : Outport  PortName=mBESS2  Element=voltage
  Out Bus Element1 : Outport  PortName=mBESS2  Element=current
  Out Bus Element2 : Outport  PortName=mBESS2  Element=active power
  Out Bus Element3 : Outport  PortName=mBESS2  Element=reactive power
  wires:
  Low-Pass Filter (Discrete or Continuous)1/1 -> Out Bus Element2/1
  Low-Pass Filter (Discrete or Continuous)/1 -> Out Bus Element3/1
  PS-Simulink Converter3/1 -> Out Bus Element1/1
  PS-Simulink Converter7/1 -> Low-Pass Filter (Discrete or Continuous)/1
  PS-Simulink Converter6/1 -> Low-Pass Filter (Discrete or Continuous)1/1
  PS-Simulink Converter2/1 -> Out Bus Element/1
  connections:
  ~/RConn1 -- Power Sensor (Three-Phase)1/RConn1
  Power Sensor (Three-Phase)1/LConn3 -- PS-Simulink Converter7/LConn1
  Power Sensor (Three-Phase)1/LConn2 -- PS-Simulink Converter6/LConn1
  Current and Voltage Sensor (Three-Phase)/RConn2 -- PS-Simulink Converter3/LConn1
  PS-Simulink Converter2/LConn1 -- Current and Voltage Sensor (Three-Phase)/RConn1
  Current and Voltage Sensor (Three-Phase)/LConn1 -- a1/RConn1
  Power Sensor (Three-Phase)1/LConn1 -- Current and Voltage Sensor (Three-Phase)/RConn3

== system IndustrialMicrogrid/MG2 Primary Substation/BESS and Controller 2/BESS output filter and transformer1 ==
  10 kvar : ee_lib/Passive/RLC Assemblies/Wye-Connected Load  parameterization=ee.enum.rlc.parameterization.ratedpower  component_structure=ee.enum.rlc.structure.C  component_structure_PQ=ee.enum.rlc.structure.C  R=1 Ohm  L=0.001 H  C=1e-6 F  VRated=microgrid.voltage V  FRated=grid.frequency Hz  P=0 W  Qpos=0 A*V  Qneg=BESS.qBESSFilter A*V  R_parasitic=1e-6 Ohm  G_parasitic=1e-6 1/Ohm  R_parasitic_PQ=1e-6 Ohm  G_parasitic_PQ=1e-6 1/Ohm  Vmag0=microgrid.voltage V  Vang0=0 deg  Freq0=grid.frequency Hz  IL_specify=on  IL_priority=High  IL=[ 0 0 0 ] A  IL_nominal_specify=off  IL_nominal_unit=A  IL_nominal_value=1  VC_specify=on  VC_priority=High  VC=[ 0 0 0 ] V  VC_nominal_specify=off  VC_nominal_unit=V  VC_nominal_value=1
  Electrical Reference1 : fl_lib/Electrical/Electrical Elements/Electrical Reference
  Transformer 1 kV/13.8 kV : Subsystem
      mask Display: image('$imagefile'); % Use "Edit Image" on toolstrip to change.
  "~ " : PMIOPort  Side=Right
  ~ : PMIOPort  Port=2  Side=Left
  connections:
  Electrical Reference1/LConn1 -- 10 kvar/RConn1
  10 kvar/LConn1 -- Transformer 1 kV/13.8 kV/RConn1 -- "~ "/RConn1
  Transformer 1 kV/13.8 kV/LConn1 -- ~/RConn1

== system IndustrialMicrogrid/MG2 Primary Substation/Microgrid Controller 2/Active and Reactive Power Reference ==
  Bus Element In3 : Inport  PortName=Control Room  Element=PlannedIslandCmd2
  Bus Element In6 : Inport  PortName=Control Room  Element=Pref2
  Bus Element In1 : Inport  PortName=Control Room  Element=Qref2
  Bus Element In5 : Inport  Port=2  PortName=MGController  Element=IslandMGController2.MGPlannedIsland2.plannedislandP
  Bus Element In4 : Inport  Port=2  PortName=MGController  Element=IslandMGController2.MGPlannedIsland2.plannedislandQ
  Mux : Mux  Inputs=2
  Saturation : Saturate  UpperLimit=PQUpperLimit  LowerLimit=PQLowerLimit
  Sum : Sum  Inputs=|++
  Sum1 : Sum  Inputs=|++
  Switch : Switch  Criteria=u2 > Threshold  Threshold=0.5  SaturateOnIntegerOverflow=off  InputSameDT=off
  Switch1 : Switch  Criteria=u2 > Threshold  Threshold=0.5  SaturateOnIntegerOverflow=off  InputSameDT=off
  PQref : Outport
  wires:
  Sum/1 -> Switch/1
  Bus Element In1/1 -> Switch1/3, Sum1/2
  Switch/1 -> Mux/1  "Pref"
  Bus Element In6/1 -> Switch/3, Sum/2
  Bus Element In4/1 -> Sum1/1
  Bus Element In3/1 -> Switch/2, Switch1/2
  Sum1/1 -> Switch1/1
  Switch1/1 -> Mux/2  "Qref"
  Saturation/1 -> PQref/1
  Bus Element In5/1 -> Sum/1
  Mux/1 -> Saturation/1  "PQref"

== system IndustrialMicrogrid/MG2 Primary Substation/Microgrid Controller 2/Black Start ==
  Bus Element In6 : Inport  PortName=Control Room  Element=VFMode2
  Bus Element In1 : Inport  PortName=Control Room  Element=Vref2
  Bus Element In2 : Inport  PortName=Control Room  Element=Fref2
  Bus Element In3 : Inport  PortName=Control Room  Element=BlackStartMG2
  Bus Element In4 : Inport  PortName=Control Room  Element=BlackStartMG2
  Constant : Constant
  If : If
  If Action Subsystem : Subsystem  TreatAsAtomicUnit=on
  If Action Subsystem1 : Subsystem  TreatAsAtomicUnit=on
  Merge : Merge
  Merge1 : Merge
  Switch : Switch  Criteria=u2 > Threshold  Threshold=0.5  SaturateOnIntegerOverflow=off  InputSameDT=off
  Bus Element Out1 : Outport  PortName=BlackStartcontroller2  Element=VFMode2
  Bus Element Out2 : Outport  PortName=BlackStartcontroller2  Element=Vref2
  Bus Element Out3 : Outport  PortName=BlackStartcontroller2  Element=Fref2
  wires:
  Bus Element In6/1 -> Switch/3
  Constant/1 -> Switch/1
  Bus Element In3/1 -> Switch/2
  Switch/1 -> Bus Element Out1/1  "VFMode2"
  Bus Element In1/1 -> If Action Subsystem1/1(Control Room)
  If/1 -> If Action Subsystem/Action
  If/2 -> If Action Subsystem1/Action
  If Action Subsystem/1(Out1) -> Merge/1
  If Action Subsystem1/1(Out1) -> Merge/2
  Bus Element In2/1 -> If Action Subsystem1/2(Control Room1)
  If Action Subsystem/2(Out2) -> Merge1/1
  If Action Subsystem1/2(Out2) -> Merge1/2
  Bus Element In4/1 -> If/1
  Merge/1 -> Bus Element Out2/1  "Vref"
  Merge1/1 -> Bus Element Out3/1  "Fref"
